simulink model "pdl_linear_hw2"  (R2017a)
settings: Solver=VariableStepAuto  StartTime=0.0  StopTime=duration  RelTol=1e-3
values from neighbouring files (symbols this model uses):
  A = [0 0 1 0; 0 0 0 1; -k/M -m*g/M -b/M 0; k/(M*L) (m+M)*g/(M*L) b/(M*L) 0]    [pendulum_hw2.m]
  B = [0;0;1/M;-1/(M*L)]    [pendulum_hw2.m]
  E = [0 0;0 0;-1/M 0;1/(M*L) -1/(m*L)]    [pendulum_hw2.m]
  f_p = 1e-4    (= 0.0001)    [pendulum_hw2.m]
  K = lqr(A,B,Q,R)    [pendulum_hw2.m]
  Nbar = -pinv(B)*A*pinv(Cn)+K*pinv(Cn)    [pendulum_hw2.m]
  Ts = 0.001    [pendulum_hw2.m]
  w_p = 10    [pendulum_hw2.m]
  X_0 = [0;1*pi/180;0;0]    [pendulum_hw2.m]
libraries: simulink x2
settings Model: Creator=Salmon  LastModifiedBy=Salmon

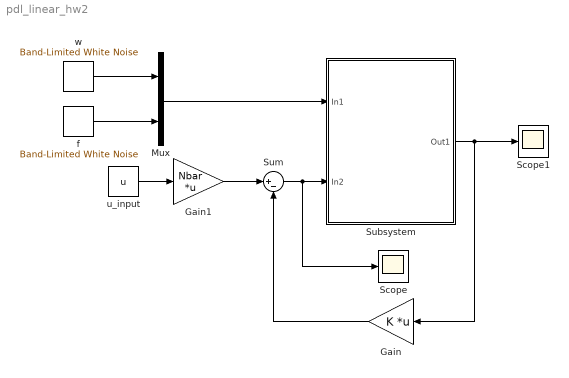
== system pdl_linear_hw2 ==
  Gain : Gain  Gain=K  Multiplication=Matrix(K*u)
  Gain1 : Gain  Gain=Nbar  Multiplication=Matrix(K*u)
  Mux : Mux  Inputs=2
  Scope : Scope
  Scope1 : Scope
  Subsystem : Subsystem
  Sum : Sum  Inputs=|+-
  f : simulink/Sources/Band-Limited White Noise  Cov=[f_p]  Ts=Ts  seed=[23341]
  u_input : Constant  Value=u
  w : simulink/Sources/Band-Limited White Noise  Cov=[w_p]  Ts=Ts  seed=[23341]
  wires:
  w/1 -> Mux/1
  f/1 -> Mux/2
  Mux/1 -> Subsystem/1(In1)
  u_input/1 -> Gain1/1
  Subsystem/1(Out1) -> Scope1/1, Gain/1
  Sum/1 -> Scope/1, Subsystem/2(In2)
  Gain/1 -> Sum/2
  Gain1/1 -> Sum/1

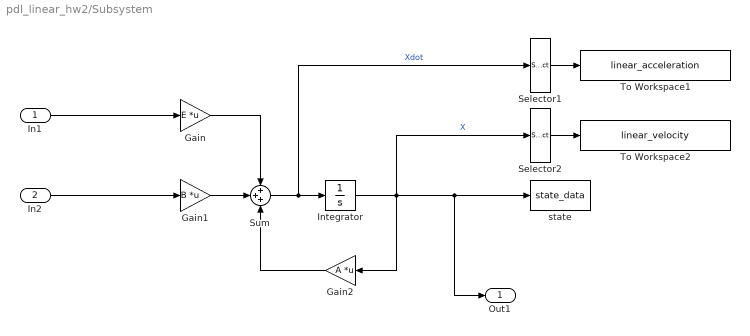
== system pdl_linear_hw2/Subsystem ==
  In1 : Inport
  In2 : Inport  Port=2
  Gain : Gain  Gain=E  Multiplication=Matrix(K*u)
  Gain1 : Gain  Gain=B  Multiplication=Matrix(K*u)
  Gain2 : Gain  Gain=A  Multiplication=Matrix(K*u)
  Integrator : Integrator  InitialCondition=X_0
  Selector1 : Selector  InputPortWidth=4  IndexOptions=Index vector (dialog)  Indices=[3]  OutputSizes=1
  Selector2 : Selector  InputPortWidth=4  IndexOptions=Index vector (dialog)  Indices=[3]  OutputSizes=1
  Sum : Sum  Inputs=+++
  To Workspace1 : ToWorkspace  VariableName=linear_acceleration  SaveFormat=Structure With Time  SampleTime=-1
  To Workspace2 : ToWorkspace  VariableName=linear_velocity  SaveFormat=Structure With Time  SampleTime=-1
  state : ToWorkspace  VariableName=state_data  SaveFormat=Structure With Time  SampleTime=Ts
  Out1 : Outport
  wires:
  In1/1 -> Gain/1
  Gain/1 -> Sum/1
  Gain1/1 -> Sum/2
  Selector2/1 -> To Workspace2/1
  Selector1/1 -> To Workspace1/1
  Gain2/1 -> Sum/3
  In2/1 -> Gain1/1
  Integrator/1 -> Gain2/1, Selector2/1, Out1/1, state/1  "X"
  Sum/1 -> Integrator/1, Selector1/1  "Xdot"
